simulink model "Sensor_fusion_Kalman_v5_R2017a"  (R2020a)
settings: Solver=FixedStepDiscrete  StartTime=0.0  StopTime=10  FixedStep=0.001  RelTol=1e-3  EnableMultiTasking=on
libraries: arduinosensorlib x1
settings Model: SILPILModeSetting=veronly  ExtModeTrigDuration=2  Creator=Roger  LastModifiedBy=InFla
settings DataIOCC: LimitDataPoints=on  SaveFormat=Array  ReturnWorkspaceOutputs=off
settings OptimizationCC: EnhancedBackFolding=on  PassReuseOutputArgsAs=Individual arguments  ZeroExternalMemoryAtStartup=off  ZeroInternalMemoryAtStartup=off  MaxStackSize=64  OptimizeBlockOrder=speed  DifferentSizesBufferReuse=on  OptimizationCustomize=off  EfficientTunableParamExpr=on
settings DebuggingCC: ParameterTunabilityLossMsg=error  SFUnexpectedBacktrackingDiag=warning  SFNoUnconditionalDefaultTransitionDiag=warning  SFExecutionAtInitializationDiag=none  ArithmeticOperatorsInVariantConditions=warning
settings HardwareCC: ProdBitPerInt=16  ProdBitPerPointer=16  ProdBitPerSizeT=16  ProdBitPerPtrDiffT=16  ProdLargestAtomicFloat=None  ProdWordSize=8  ProdHWDeviceType=Atmel->AVR  UseEmbeddedCoderFeatures=off  UseSimulinkCoderFeatures=off
settings ModelReferenceCC: PropagateSignalLabelsOutOfModel=off
settings SFSimCC: SimUseLocalCustomCode=off  MATLABDynamicMemAlloc=off  CustomCodeUndefinedFunction=UseInterfaceOnly
settings RTWCC: SystemTargetFile=ert.tlc  HardwareBoard=Arduino Uno  TLCOptions=-aInlineSetEventsForThisBaseRateFcn=TLC_FALSE -aSuppressMultiTaskScheduler=TLC_FALSE -aRateBasedStepFcn=1  TemplateMakefile=ert_default_tmf  RTWUseLocalCustomCode=off  Toolchain=Arduino AVR  BuildConfiguration=Faster Runs
settings CodeAppCC: ForceParamTrailComments=on  IgnoreCustomStorageClasses=off  OperatorAnnotations=on  SimulinkDataObjDesc=on  SFDataObjDesc=on  InsertBlockDesc=on
settings ERTTargetCC: SupportContinuousTime=on  SupportNonInlinedSFcns=on  SupportVariableSizeSignals=on  ExtModeStaticAllocSize=250
settings ConfigComp: CovMetricSettings=dw  CovHtmlReporting=on  CovSaveCumulativeToWorkspaceVar=on  CovSaveSingleToWorkspaceVar=on  CovExternalEMLEnable=off

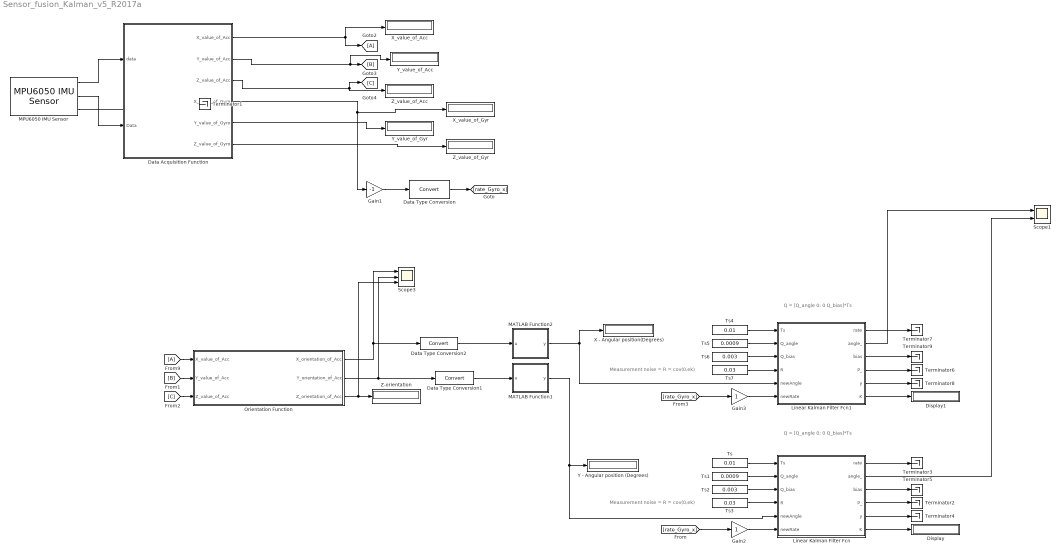
== system Sensor_fusion_Kalman_v5_R2017a ==
  note: Measurement noise = R = cov(0,ek)
  note: Q = [Q_angle 0; 0 Q_bias]*Ts
  note: Measurement noise = R = cov(0,ek)
  note: Q = [Q_angle 0; 0 Q_bias]*Ts
  Data Acquisition Function : MATLAB Function  TreatAsAtomicUnit=on
  Data Type Conversion : DataTypeConversion
  Data Type Conversion1 : DataTypeConversion
  Data Type Conversion2 : DataTypeConversion
  Display : Display
  Display1 : Display
  Gain1 : Gain  Gain=-1
  Gain2 : Gain
  Gain3 : Gain
  Linear Kalman Filter Fcn : MATLAB Function  TreatAsAtomicUnit=on
  Linear Kalman Filter Fcn1 : MATLAB Function  TreatAsAtomicUnit=on
  MATLAB Function1 : MATLAB Function  TreatAsAtomicUnit=on
  MATLAB Function2 : MATLAB Function  TreatAsAtomicUnit=on
  MPU6050 IMU Sensor : arduinosensorlib/MPU6050 IMU Sensor  SlaveAddress=0x68  Accel=on  AngularRate=on  Temperature=off  Status=on  EulerAngles=off  Quat=off  AccelRange=2G  GyroRange=250 dps  DmpOdr=200 Hz  Dlpf=Accelerometer: 184Hz, Gyroscope: 188Hz  SampleTime=0.05
      settings: SourceProductBaseCode=ARDUINO
  Orientation Function : MATLAB Function  TreatAsAtomicUnit=on
  Scope1 : Scope  NumInputPorts=2
  Scope3 : Scope  NumInputPorts=3
  Terminator{1..9} (9 alike) : Terminator
  Ts : Constant  Value=0.01
  Ts1 : Constant  Value=0.0009
  Ts2 : Constant  Value=0.003
  Ts3 : Constant  Value=0.03
  Ts4 : Constant  Value=0.01
  Ts5 : Constant  Value=0.0009
  Ts6 : Constant  Value=0.003
  Ts7 : Constant  Value=0.03
  X - Angular position(Degrees) : Display
  X_value_of_Acc : Display
      settings: Format=bank
  X_value_of_Gyr : Display
      settings: Format=bank
  Y - Angular position (Degrees) : Display
  Y_value_of_Acc : Display
      settings: Format=bank
  Y_value_of_Gyr : Display
      settings: Format=bank
  Z-orientation : Display
      settings: Format=bank
  Z_value_of_Acc : Display
      settings: Format=bank
  Z_value_of_Gyr : Display
      settings: Format=bank
  wires:
  Orientation Function/1(X_orientation_of_Acc) -> Scope3/1, Data Type Conversion2/1
  [A] -> Orientation Function/1(X_value_of_Acc)
  Gain1/1 -> Data Type Conversion/1
  MPU6050 IMU Sensor/3 -> Terminator1/1
  Data Type Conversion1/1 -> MATLAB Function1/1(u)
  Data Type Conversion/1 -> [rate_Gyro_x]
  MATLAB Function1/1(y) -> Linear Kalman Filter Fcn/5(newAngle), Y - Angular position (Degrees)/1
  [rate_Gyro_x] -> Gain2/1
  Orientation Function/2(Y_orientation_of_Acc) -> Data Type Conversion1/1, Scope3/2
  Ts3/1 -> Linear Kalman Filter Fcn/4(R)
  Ts/1 -> Linear Kalman Filter Fcn/1(Ts)
  Ts1/1 -> Linear Kalman Filter Fcn/2(Q_angle)
  Ts2/1 -> Linear Kalman Filter Fcn/3(Q_bias)
  Gain2/1 -> Linear Kalman Filter Fcn/6(newRate)
  Orientation Function/3(Z_orientation_of_Acc) -> Scope3/3, Z-orientation/1
  [B] -> Orientation Function/2(Y_value_of_Acc)
  [C] -> Orientation Function/3(Z_value_of_Acc)
  Linear Kalman Filter Fcn/5(y) -> Terminator4/1
  Linear Kalman Filter Fcn/4(P_) -> Terminator2/1
  Linear Kalman Filter Fcn/3(bias) -> Terminator5/1
  Linear Kalman Filter Fcn/1(rate) -> Terminator3/1
  Linear Kalman Filter Fcn/2(angle_) -> Scope1/2
  Linear Kalman Filter Fcn/6(K) -> Display/1
  MPU6050 IMU Sensor/1 -> Data Acquisition Function/1(data)
  MPU6050 IMU Sensor/2 -> Data Acquisition Function/2(Data)
  Data Type Conversion2/1 -> MATLAB Function2/1(u)
  Linear Kalman Filter Fcn1/2(angle_) -> Scope1/1
  Linear Kalman Filter Fcn1/6(K) -> Display1/1
  Ts5/1 -> Linear Kalman Filter Fcn1/2(Q_angle)
  MATLAB Function2/1(y) -> Linear Kalman Filter Fcn1/5(newAngle), X - Angular position(Degrees)/1
  Linear Kalman Filter Fcn1/4(P_) -> Terminator6/1
  Linear Kalman Filter Fcn1/5(y) -> Terminator8/1
  Linear Kalman Filter Fcn1/3(bias) -> Terminator9/1
  Linear Kalman Filter Fcn1/1(rate) -> Terminator7/1
  Ts4/1 -> Linear Kalman Filter Fcn1/1(Ts)
  Ts6/1 -> Linear Kalman Filter Fcn1/3(Q_bias)
  Gain3/1 -> Linear Kalman Filter Fcn1/6(newRate)
  [rate_Gyro_x] -> Gain3/1
  Ts7/1 -> Linear Kalman Filter Fcn1/4(R)
  Data Acquisition Function/5(Y_value_of_Gyro) -> Y_value_of_Gyr/1
  Data Acquisition Function/1(X_value_of_Acc) -> [A], X_value_of_Acc/1
  Data Acquisition Function/2(Y_value_of_Acc) -> Y_value_of_Acc/1, [B]
  Data Acquisition Function/3(Z_value_of_Acc) -> Z_value_of_Acc/1, [C]
  Data Acquisition Function/4(X_value_of_Gyro) -> X_value_of_Gyr/1, Gain1/1
  Data Acquisition Function/6(Z_value_of_Gyro) -> Z_value_of_Gyr/1

== matlab function Sensor_fusion_Kalman_v5_R2017a/MATLAB Function1 ==
  data: u input; y output
function y = fcn(u)

if(isnan(u))
y=0;
else
y=u;
end

== matlab function Sensor_fusion_Kalman_v5_R2017a/Linear Kalman Filter Fcn ==
  data: Ts input; Q_angle input; Q_bias input; R input; newAngle input; rate output; newRate input; angle_ output; bias output; P_ output; y output; K output
% Algorithm -- implimentation of Linear-Kalman filter for a 6-DOF IMU using
% a single axis for testing. A single axis consisting of both anaccelerometer
% input and gyroscope input from IMU.
% Author: RM van Rensburg
% for IMU testing purposes
% Date: 26-04-2015
% Version: 1.0,tested on Matlab R2015a

function [rate,angle_,bias,P_,y,K] = Kalmanf(Ts,...
                                             Q_angle,Q_bias,R,...
                                             newAngle,...
                                             newRate)
                      
% Process noise covariance matrix  
Q = [Q_angle 0;0 Q_bias]*Ts;
A = [1  -Ts;0  1];
C = [1 0];
bias = 0.0;

rate = newRate - bias;

persistent angle;
if isempty(angle);angle = 0;
else angle = angle + (Ts * rate); 
end
angle_= angle;
                    
persistent P;
if isempty(P);P = [0 0 ; 0 0]; 
else P = A*P*A' + Q;
end
P_=P;

S = C*P*C' + R; % Estimate error 
K = (P_*C')/S; % Kalman gain
y = newAngle - angle_; % Angle difference 
xk = angle_ + K*y;
angle_ = xk(1);
bias = xk(2);
angle = angle_;

% Update the error covariance 
I = [1 0;0 1];
P_ = (I - K*C)*P_;
% or
% Joseph form (more stable)
% P_ = (I - K*C)*P_*(I - K*C) + K*R*K';
P = P_;

return

end

== matlab function Sensor_fusion_Kalman_v5_R2017a/Linear Kalman Filter Fcn1 ==
  data: Ts input; Q_angle input; Q_bias input; R input; newAngle input; rate output; newRate input; angle_ output; bias output; P_ output; y output; K output
% Algorithm -- implimentation of Linear-Kalman filter for a 6-DOF IMU using
% a single axis for testing. A single axis consisting of both anaccelerometer
% input and gyroscope input from IMU.
% Author: RM van Rensburg
% for IMU testing purposes
% Date: 26-04-2015
% Version: 1.0,tested on Matlab R2015a

function [rate,angle_,bias,P_,y,K] = Kalmanf(Ts,...
                                             Q_angle,Q_bias,R,...
                                             newAngle,...
                                             newRate)
                      
% Process noise covariance matrix  
Q = [Q_angle 0;0 Q_bias]*Ts;
A = [1  -Ts;0  1];
C = [1 0];
bias = 0.0;

rate = newRate - bias;

persistent angle;
if isempty(angle);angle = 0;
else angle = angle + (Ts * rate); 
end
angle_= angle;
                    
persistent P;
if isempty(P);P = [0 0 ; 0 0]; 
else P = A*P*A' + Q;
end
P_=P;

S = C*P*C' + R; % Estimate error 
K = (P_*C')/S; % Kalman gain
y = newAngle - angle_; % Angle difference 
xk = angle_ + K*y;
angle_ = xk(1);
bias = xk(2);
angle = angle_;

% Update the error covariance 
I = [1 0;0 1];
P_ = (I - K*C)*P_;
% or
% Joseph form (more stable)
% P_ = (I - K*C)*P_*(I - K*C) + K*R*K';
P = P_;

return

end

== matlab function Sensor_fusion_Kalman_v5_R2017a/Data Acquisition Function ==
  data: data input; Data input; X_value_of_Acc output; Y_value_of_Acc output; Z_value_of_Acc output; X_value_of_Gyro output; Y_value_of_Gyro output; Z_value_of_Gyro output
% Reading IMU packet bytes from Sensor Stream App 
% Author: RM van Rensburg
% Date: 26-04-2015
% Version: 1.0,tested on Matlab R2015a

function [X_value_of_Acc,Y_value_of_Acc, Z_value_of_Acc,...
          X_value_of_Gyro, Y_value_of_Gyro, Z_value_of_Gyro]...
          = fcn(data, Data)
             
% Header packet
% Header = Data(1:4);

% Accelerometer data
X_value_of_Acc = data(1,:);
Y_value_of_Acc = data(2,:);
Z_value_of_Acc = data(3,:);

% Gyroscope data
X_value_of_Gyro = Data(1,:);
Y_value_of_Gyro = Data(2,:);
Z_value_of_Gyro = Data(3,:);

% Proximity sensor
% X_value_of_Tes = typecast(uint8(Data(29:36)),'double');
% Y_value_of_Tes = typecast(uint8(Data(37:44)),'double');
% Z_value_of_Tes = typecast(uint8(Data(45:52)),'double');

== matlab function Sensor_fusion_Kalman_v5_R2017a/MATLAB Function2 ==
  data: u input; y output
function y = fcn(u)

if(isnan(u))
y=0;
else
y=u;
end

== matlab function Sensor_fusion_Kalman_v5_R2017a/Orientation Function ==
  data: X_value_of_Acc input; X_orientation_of_Acc output; Y_orientation_of_Acc output; Z_orientation_of_Acc output; Y_value_of_Acc input; Z_value_of_Acc input
% Computing orientation of tri-axial acclerometer data from IMU 
% Author: RM van Rensburg
% Date: 26-04-2015
% Version: 1.0,tested on Matlab R2015a

function [X_orientation_of_Acc,...
          Y_orientation_of_Acc,...
          Z_orientation_of_Acc]...
          = OrientationFcn(X_value_of_Acc,Y_value_of_Acc,Z_value_of_Acc)
     
      
% Using x and y from accelerometer (g-forces), calculate x and y angles
% Data directly obtained from IMU
% Using the following formulae
% Ax = arctan{X/sqrt(Y*Y + Z*Z)}
% Ay = arctan{Y/sqrt(X*X + Z*Z)}

% Computing the X*X, Y*Y, Z*Z
X2 = power(X_value_of_Acc,2);
Y2 = power(Y_value_of_Acc,2);
Z2 = power(Z_value_of_Acc,2);

% x-axis angle
result = sqrt(Y2 + Z2);
result = X_value_of_Acc / result;
x_angle_rad = atan(result);
X_orientation_of_Acc = (x_angle_rad * 180) / pi;

% y-axis angle
result = sqrt(X2 + Z2);
result = Y_value_of_Acc / result;
y_angle_rad = atan(result);
Y_orientation_of_Acc = (y_angle_rad * 180) / pi;

% z-axis angle
result = sqrt(Y2 + X2);
result = Z_value_of_Acc / result;
z_angle_rad = atan(result);
Z_orientation_of_Acc = (z_angle_rad * 180) / pi;

end
